simulink model "model"  (R2023a)
settings: Solver=VariableStepAuto  StartTime=0.0  StopTime=50  RelTol=1e-6
values from neighbouring files (symbols this model uses):
  ParSt = MyObject    [main.m]
  ParUnst = MyObject    [main.m]
settings Model: Creator=User  LastModifiedBy=Константин

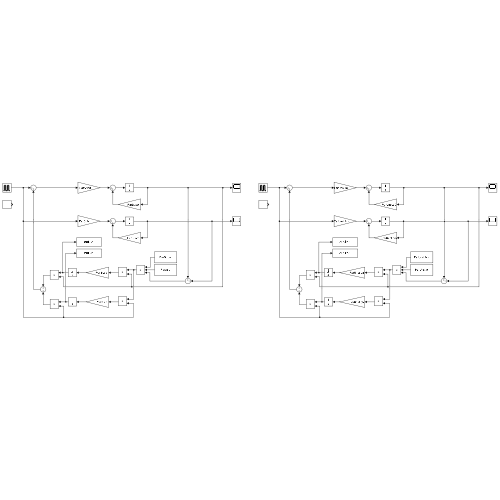
[thumbnail: Simulink's stored preview of the top-level diagram]
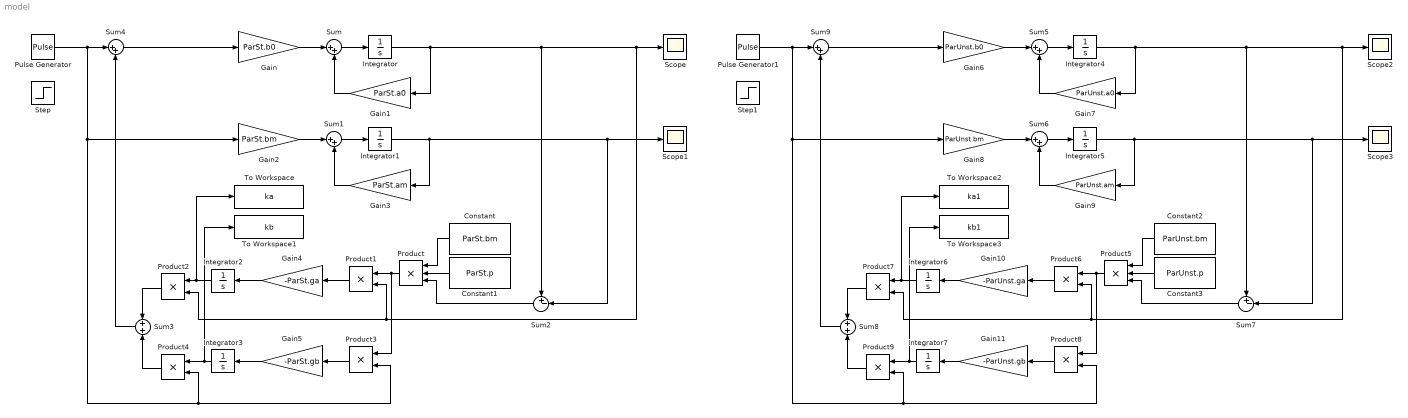
== system model ==
  Constant : Constant  Value=ParSt.bm
  Constant1 : Constant  Value=ParSt.p
  Constant2 : Constant  Value=ParUnst.bm
  Constant3 : Constant  Value=ParUnst.p
  Gain : Gain  Gain=ParSt.b0
  Gain1 : Gain  Gain=ParSt.a0
  Gain10 : Gain  Gain=-ParUnst.ga
  Gain11 : Gain  Gain=-ParUnst.gb
  Gain2 : Gain  Gain=ParSt.bm
  Gain3 : Gain  Gain=ParSt.am
  Gain4 : Gain  Gain=-ParSt.ga
  Gain5 : Gain  Gain=-ParSt.gb
  Gain6 : Gain  Gain=ParUnst.b0
  Gain7 : Gain  Gain=ParUnst.a0
  Gain8 : Gain  Gain=ParUnst.bm
  Gain9 : Gain  Gain=ParUnst.am
  Integrator{,1..7} (8 alike) : Integrator
  Product : Product  Inputs=3
  Product{1..4,6..9} (8 alike) : Product
  Product5 : Product  Inputs=3
  Pulse Generator : DiscretePulseGenerator  PulseType=Time based  Period=20  PulseWidth=50
  Pulse Generator1 : DiscretePulseGenerator  PulseType=Time based  Period=20  PulseWidth=50
  Scope{,1..3} (4 alike) : Scope
  Step : Step  Time=0  SampleTime=0
  Step1 : Step  Time=0  SampleTime=0
  Sum{,1,4..6,9} (6 alike) : Sum  Inputs=|++
  Sum2 : Sum  Inputs=+-|
  Sum3 : Sum
  Sum7 : Sum  Inputs=+-|
  Sum8 : Sum
  To Workspace : ToWorkspace  VariableName=ka  SaveFormat=Structure With Time  SampleTime=-1
  To Workspace1 : ToWorkspace  VariableName=kb  SaveFormat=Structure With Time  SampleTime=-1
  To Workspace2 : ToWorkspace  VariableName=ka1  SaveFormat=Structure With Time  SampleTime=-1
  To Workspace3 : ToWorkspace  VariableName=kb1  SaveFormat=Structure With Time  SampleTime=-1
  wires:
  Sum/1 -> Integrator/1
  Integrator/1 -> Product1/2, Product2/2, Scope/1, Sum2/1, Gain1/1
  Gain1/1 -> Sum/2
  Gain/1 -> Sum/1
  Gain2/1 -> Sum1/1
  Gain3/1 -> Sum1/2
  Integrator1/1 -> Sum2/2, Scope1/1, Gain3/1
  Sum1/1 -> Integrator1/1
  Constant/1 -> Product/1
  Constant1/1 -> Product/2
  Sum2/1 -> Product/3
  Product/1 -> Product3/1, Product1/1
  Product1/1 -> Gain4/1
  Gain4/1 -> Integrator2/1
  Integrator2/1 -> To Workspace/1, Product2/1
  Product3/1 -> Gain5/1
  Gain5/1 -> Integrator3/1
  Integrator3/1 -> To Workspace1/1, Product4/1
  Product2/1 -> Sum3/1
  Sum4/1 -> Gain/1
  Sum3/1 -> Sum4/2
  Product4/1 -> Sum3/2
  Pulse Generator/1 -> Product3/2, Product4/2, Gain2/1, Sum4/1
  Integrator7/1 -> To Workspace3/1, Product9/1
  Sum8/1 -> Sum9/2
  Integrator6/1 -> To Workspace2/1, Product7/1
  Sum9/1 -> Gain6/1
  Product9/1 -> Sum8/2
  Product8/1 -> Gain11/1
  Gain7/1 -> Sum5/2
  Constant3/1 -> Product5/2
  Gain10/1 -> Integrator6/1
  Product7/1 -> Sum8/1
  Sum7/1 -> Product5/3
  Gain11/1 -> Integrator7/1
  Sum5/1 -> Integrator4/1
  Product6/1 -> Gain10/1
  Integrator5/1 -> Sum7/2, Scope3/1, Gain9/1
  Gain8/1 -> Sum6/1
  Constant2/1 -> Product5/1
  Sum6/1 -> Integrator5/1
  Gain9/1 -> Sum6/2
  Product5/1 -> Product8/1, Product6/1
  Integrator4/1 -> Product6/2, Product7/2, Scope2/1, Sum7/1, Gain7/1
  Pulse Generator1/1 -> Product8/2, Product9/2, Gain8/1, Sum9/1
  Gain6/1 -> Sum5/1
